simulink model "kingtaha1"  (R2022a)
settings: Solver=VariableStepAuto  StartTime=0.0  StopTime=10.0  RelTol=1e-3
settings Model: Creator=victus-pc  LastModifiedBy=victus-pc

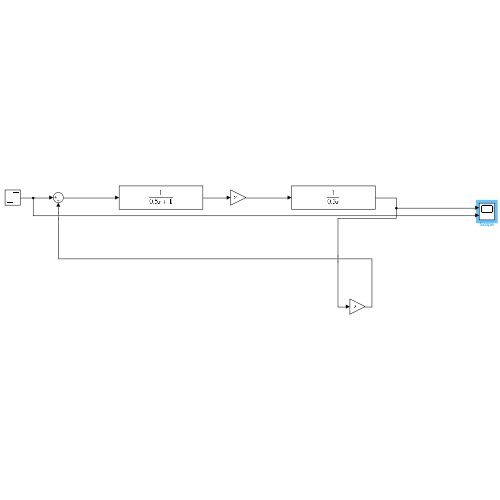
[thumbnail: Simulink's stored preview of the top-level diagram]
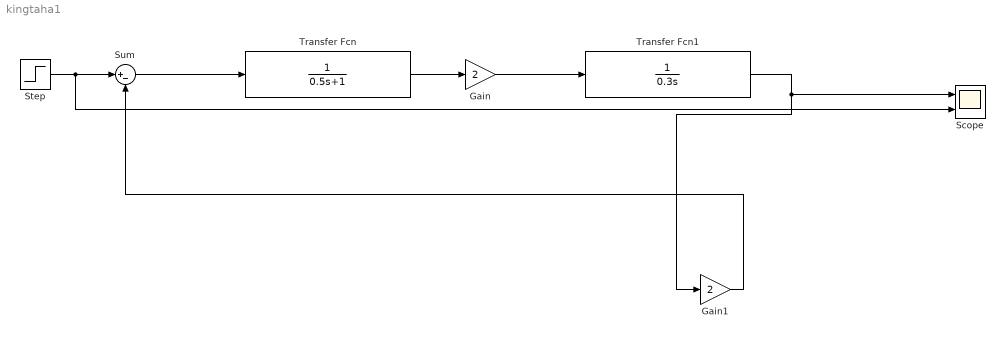
== system kingtaha1 ==
  Gain : Gain  Gain=2
  Gain1 : Gain  Gain=2
  Scope : Scope  NumInputPorts=2
  Step : Step  Time=0  SampleTime=0
  Sum : Sum  Inputs=|+-
  Transfer Fcn : TransferFcn  Denominator=[0.5 1]
  Transfer Fcn1 : TransferFcn  Denominator=[0.3 0]
  wires:
  Sum/1 -> Transfer Fcn/1
  Transfer Fcn/1 -> Gain/1
  Gain/1 -> Transfer Fcn1/1
  Transfer Fcn1/1 -> Gain1/1, Scope/1
  Gain1/1 -> Sum/2
  Step/1 -> Scope/2, Sum/1
